simulink model "ILCUpdate_th"  (R2018a)
settings: Solver=FixedStepAuto  StartTime=0.0  StopTime=20  FixedStep=sm.Ts  RelTol=1e-3
undefined symbols (not defined in the file or in its folder): get, hot
libraries: determineIterationPhase_ul x1, determineSimulationPhase_ul x1, ILCUpdate x1, dspsnks4 x1
settings Model: Creator=mitch  LastModifiedBy=mitch

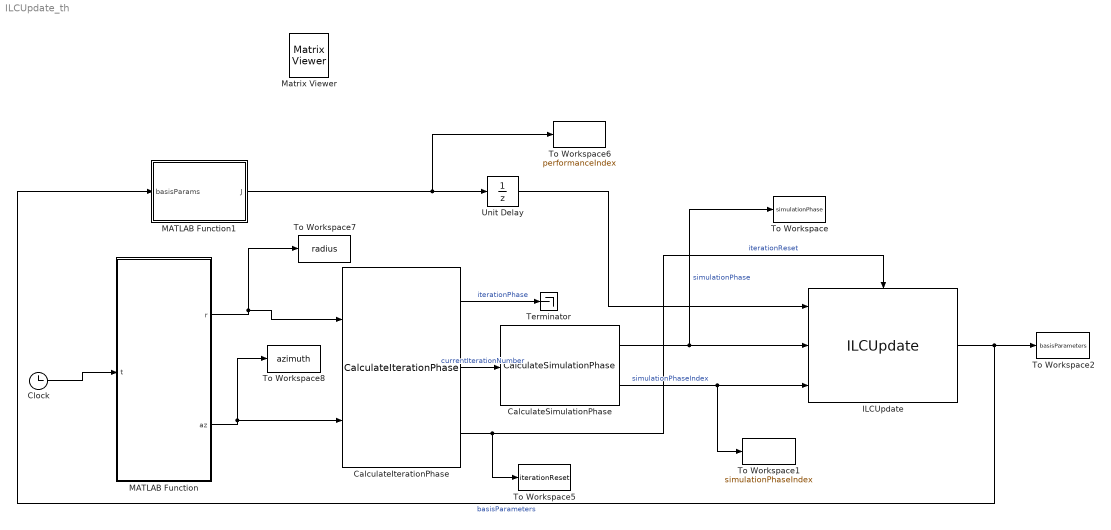
== system ILCUpdate_th ==
  CalculateIterationPhase : determineIterationPhase_ul/CalculateIterationPhase
  CalculateSimulationPhase : determineSimulationPhase_ul/CalculateSimulationPhase
  Clock : Clock
  ILCUpdate : ILCUpdate/ILCUpdate
  MATLAB Function : MATLAB Function  TreatAsAtomicUnit=on
  MATLAB Function1 : MATLAB Function  TreatAsAtomicUnit=on
  Terminator : Terminator
  To Workspace : ToWorkspace  VariableName=simulationPhase  SaveFormat=Timeseries  SampleTime=-1
  To Workspace1 : ToWorkspace  VariableName=simulationPhaseIndex  SaveFormat=Timeseries  SampleTime=-1
  To Workspace2 : ToWorkspace  VariableName=basisParameters  SaveFormat=Timeseries  SampleTime=-1
  To Workspace5 : ToWorkspace  VariableName=iterationReset  SaveFormat=Timeseries  SampleTime=-1
  To Workspace6 : ToWorkspace  VariableName=performanceIndex  SaveFormat=Timeseries  SampleTime=-1
  To Workspace7 : ToWorkspace  VariableName=radius  SaveFormat=Timeseries  SampleTime=-1
  To Workspace8 : ToWorkspace  VariableName=azimuth  SaveFormat=Timeseries  SampleTime=-1
  Unit Delay : UnitDelay  SampleTime=-1
  Matrix Viewer : dspsnks4/Matrix Viewer  IOType=viewer  ImageParams=off  CMapStr=hot(256)  AxisColorbar=on  AxisParams=off  AxisOrigin=Upper left corner  AxisTickMode=Auto  XTickRange=[0 1]  YTickRange=[0 1]  XLabel=X-axis  YLabel=Y-axis  ZLabel=Z-axis  FigPos=get(0,'defaultfigureposition')  AxisZoom=off
      settings: SourceProductName=DSP System Toolbox  SourceProductBaseCode=DS  YMin=-1.0  YMax=1.0
  wires:
  Clock/1 -> MATLAB Function/1(t)
  CalculateIterationPhase/2 -> CalculateSimulationPhase/1  "currentIterationNumber"
  CalculateSimulationPhase/1 -> ILCUpdate/2, To Workspace/1  "simulationPhase"
  CalculateIterationPhase/1 -> Terminator/1  "iterationPhase"
  CalculateIterationPhase/3 -> To Workspace5/1, ILCUpdate/Trigger  "iterationReset"
  CalculateSimulationPhase/2 -> ILCUpdate/3, To Workspace1/1  "simulationPhaseIndex"
  ILCUpdate/1 -> MATLAB Function1/1(basisParams), To Workspace2/1  "basisParameters"
  MATLAB Function/2(az) -> To Workspace8/1, CalculateIterationPhase/2
  MATLAB Function/1(r) -> To Workspace7/1, CalculateIterationPhase/1
  MATLAB Function1/1(J) -> To Workspace6/1, Unit Delay/1
  Unit Delay/1 -> ILCUpdate/1

== matlab function ILCUpdate_th/MATLAB Function1 ==
  data: basisParams input; J output
function J = fcn(basisParams)

J = 100000 - 100000*(basisParams(1)-90*pi/180)^2 - 100000*(basisParams(2)-60*pi/180)^2;

end

== matlab function ILCUpdate_th/MATLAB Function ==
  data: r output; t input; az output
function [r,az] = fcn(t)

r = 70+35*sin(2*pi*t);
az = cos(2*pi*t);
end
